simulink model "parkingValetVPP"  (R2023a)
settings: Solver=VariableStepAuto  StartTime=0.0  StopTime=Duration  RelTol=1e-3
values from neighbouring files (symbols this model uses):
  Duration = 15    [ParkingValetUsingNonlinearModelPredictiveControl1.m]
  egoTargetPose = [27.2,4.7,-pi/2]    [ParkingValetUsingNonlinearModelPredictiveControl1.m]
  pTracking = 10    [ParkingValetUsingNonlinearModelPredictiveControl1.m]
  tmax = tmin + 0.5    (= 5.5)    [ParkingValetUsingNonlinearModelPredictiveControl1.m]
  tmin = 5    [ParkingValetUsingNonlinearModelPredictiveControl1.m]
  Ts = 0.1    [ParkingValetUsingNonlinearModelPredictiveControl1.m]    (also in createMPCForTrackingVPP.m)
  TsPlanner = 1    [ParkingValetUsingNonlinearModelPredictiveControl1.m]
libraries: simulink x2, mpclib x1, robotmobilelib x1, mpcadaslib x1
settings Model: Creator=The MathWorks, Inc.  LastModifiedBy=The MathWorks, Inc.
settings SolverCC: MaxZcPerStep=1
settings OptimizationCC: ReuseModelBlockBuffer=off
settings ModelReferenceCC: EnableRefExpFcnMdlSchedulingChecks=on

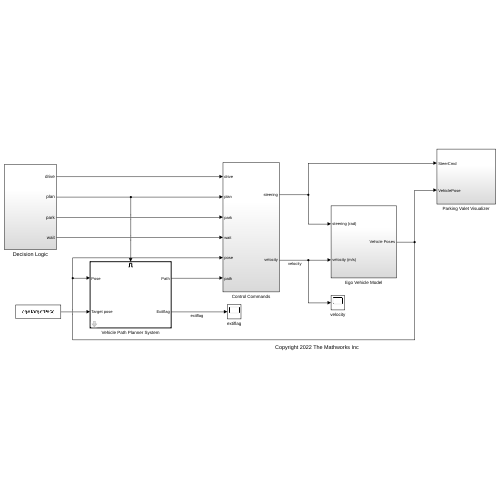
[thumbnail: Simulink's stored preview of the top-level diagram]
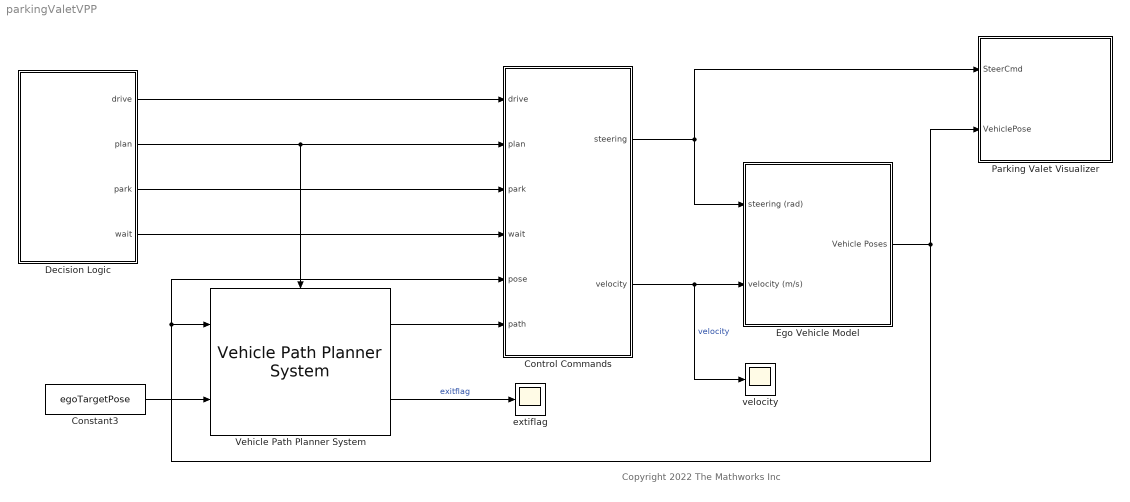
== system parkingValetVPP ==
  note: Copyright 2022 The Mathworks Inc
  Constant3 : Constant  Value=egoTargetPose
  Control Commands : Subsystem
  Decision Logic : Subsystem
  Ego Vehicle Model : Subsystem
  Parking Valet Visualizer : Subsystem
  Vehicle Path Planner System : mpcadaslib/Vehicle Path Planner System  egoLength=vdims.Length  egoWidth=vdims.Width  wheelbase=egoWheelbase  dist2Center=distToCenter  numObs=numObs  obsMat=obsMat  obs_ext=off  minDist=d_safe  Ts=TsPlanner  pPlanning=pPlanner  v_range=v_range  v_ext=off  steer_range=steer_range  steer_ext=off  suboptimal=off  maxiter=200  output_exitflag=on
      settings: LibrarySourceBlock=mpclib/Automated Driving/Vehicle Path Planner System
  extiflag : Scope
  velocity : Scope
  wires:
  Ego Vehicle Model/1(Vehicle Poses) -> Parking Valet Visualizer/2(VehiclePose), Control Commands/5(pose), Vehicle Path Planner System/1
  Control Commands/2(velocity) -> velocity/1, Ego Vehicle Model/2(velocity (m/s))  "velocity"
  Control Commands/1(steering) -> Ego Vehicle Model/1(steering (rad)), Parking Valet Visualizer/1(SteerCmd)
  Decision Logic/1(drive) -> Control Commands/1(drive)
  Decision Logic/2(plan) -> Vehicle Path Planner System/Enable, Control Commands/2(plan)
  Decision Logic/3(park) -> Control Commands/3(park)
  Decision Logic/4(wait) -> Control Commands/4(wait)
  Vehicle Path Planner System/1 -> Control Commands/6(path)
  Vehicle Path Planner System/2 -> extiflag/1  "exitflag"
  Constant3/1 -> Vehicle Path Planner System/2

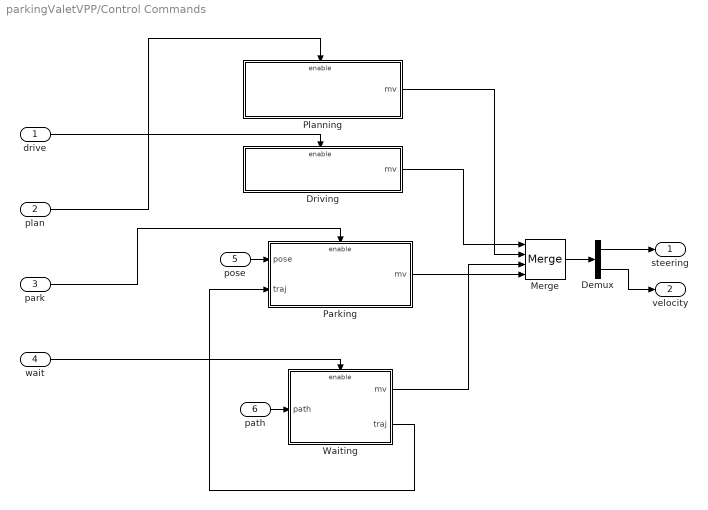
== system parkingValetVPP/Control Commands ==
  drive : Inport
  plan : Inport  Port=2
  park : Inport  Port=3
  wait : Inport  Port=4
  pose : Inport  Port=5
  path : Inport  Port=6
  Demux : Demux  Outputs=2
  Driving : Subsystem  TreatAsAtomicUnit=on
  Merge : Merge  Inputs=4
  "Parking " : Subsystem  TreatAsAtomicUnit=on
  Planning : Subsystem  TreatAsAtomicUnit=on
  Waiting : Subsystem  TreatAsAtomicUnit=on
  steering : Outport
  velocity : Outport  Port=2
  wires:
  "Parking "/1(mv) -> Merge/4
  Waiting/1(mv) -> Merge/3
  Merge/1 -> Demux/1
  Driving/1(mv) -> Merge/1
  pose/1 -> "Parking "/1(pose)
  drive/1 -> Driving/Enable
  Planning/1(mv) -> Merge/2
  Waiting/2(traj) -> "Parking "/2(traj)
  wait/1 -> Waiting/Enable
  path/1 -> Waiting/1(path)
  plan/1 -> Planning/Enable
  Demux/2 -> velocity/1
  park/1 -> "Parking "/Enable
  Demux/1 -> steering/1

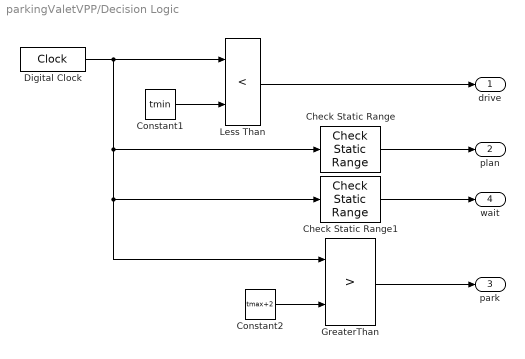
== system parkingValetVPP/Decision Logic ==
  Check Static Range : simulink/Model Verification/Check  Static Range  Description=tmin <= u <= tmax  max=tmax  max_included=on  min=tmin  min_included=on  enabled=off  stopWhenAssertionFail=off  export=on  icon=graphic
  Check Static Range1 : simulink/Model Verification/Check  Static Range  Description=tmax < u <= tmax+2  max=tmax+2  max_included=on  min=tmax  min_included=off  enabled=off  stopWhenAssertionFail=off  export=on  icon=graphic
  Constant1 : Constant  Value=tmin
  Constant2 : Constant  Value=tmax+2
  Digital Clock : DigitalClock  SampleTime=0.1
  GreaterThan : RelationalOperator  Operator=>  OutDataTypeStr=boolean  RndMeth=Simplest  InputSameDT=off
  Less Than : RelationalOperator  Operator=<  OutDataTypeStr=boolean  RndMeth=Simplest  InputSameDT=off
  drive : Outport
  plan : Outport  Port=2
  park : Outport  Port=3
  wait : Outport  Port=4
  wires:
  Constant1/1 -> Less Than/2
  Digital Clock/1 -> Check Static Range1/1, GreaterThan/1, Check Static Range/1, Less Than/1
  Constant2/1 -> GreaterThan/2
  GreaterThan/1 -> park/1
  Less Than/1 -> drive/1
  Check Static Range/1 -> plan/1
  Check Static Range1/1 -> wait/1

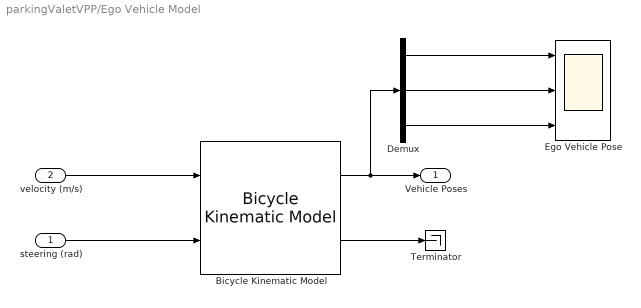
== system parkingValetVPP/Ego Vehicle Model ==
  steering (rad) : Inport
  velocity (m/s) : Inport  Port=2
  Bicycle Kinematic Model : robotmobilelib/Bicycle Kinematic Model  VehicleInputs=Vehicle Speed & Steering Angle  WheelBase=2.8  VehicleSpeedRange=[-6.5 6.5]  MaxSteeringAngle=pi/4  InitialState=egoInitialPose  SimulateUsing=Interpreted execution
  Demux : Demux  Outputs=3
  Ego Vehicle Pose : Scope  NumInputPorts=3
  Terminator : Terminator
  Vehicle Poses : Outport
  wires:
  Bicycle Kinematic Model/1 -> Demux/1, Vehicle Poses/1
  velocity (m/s)/1 -> Bicycle Kinematic Model/1
  steering (rad)/1 -> Bicycle Kinematic Model/2
  Bicycle Kinematic Model/2 -> Terminator/1
  Demux/3 -> Ego Vehicle Pose/3
  Demux/2 -> Ego Vehicle Pose/2
  Demux/1 -> Ego Vehicle Pose/1

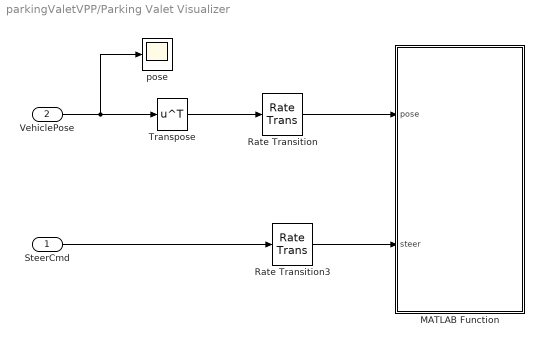
== system parkingValetVPP/Parking Valet Visualizer ==
  SteerCmd : Inport
  VehiclePose : Inport  Port=2
  MATLAB Function : MATLAB Function  TreatAsAtomicUnit=on
  Rate Transition : RateTransition  OutPortSampleTime=Tv
  Rate Transition3 : RateTransition  OutPortSampleTime=Tv
  Transpose : Math  Operator=transpose
  pose : Scope
  wires:
  Rate Transition/1 -> MATLAB Function/1(pose)
  VehiclePose/1 -> pose/1, Transpose/1
  Rate Transition3/1 -> MATLAB Function/2(steer)
  SteerCmd/1 -> Rate Transition3/1
  Transpose/1 -> Rate Transition/1

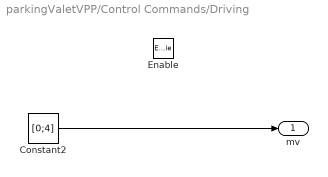
== system parkingValetVPP/Control Commands/Driving ==
  Enable : EnablePort  StatesWhenEnabling=reset
  Constant2 : Constant  Value=[0;4]  VectorParams1D=off
  mv : Outport
  wires:
  Constant2/1 -> mv/1

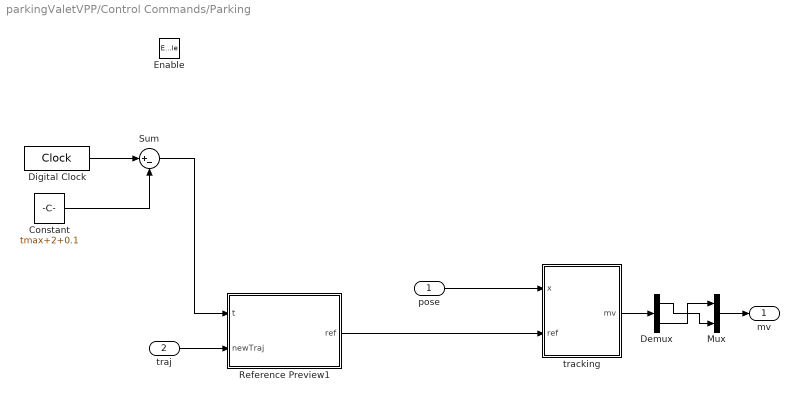
== system parkingValetVPP/Control Commands/Parking  ==
  pose : Inport
  traj : Inport  Port=2
  Enable : EnablePort  StatesWhenEnabling=reset
  Constant : Constant  Value=tmax+2+0.1
  Demux : Demux  Outputs=2
  Digital Clock : DigitalClock  SampleTime=0.1
  Mux : Mux  Inputs=2
  Reference Preview1 : MATLAB Function  TreatAsAtomicUnit=on
  Sum : Sum  Inputs=|+-
  tracking : Subsystem
  mv : Outport
  wires:
  Reference Preview1/1(ref) -> tracking/2(ref)
  pose/1 -> tracking/1(x)
  tracking/1(mv) -> Demux/1
  Demux/2 -> Mux/1
  Demux/1 -> Mux/2
  Mux/1 -> mv/1
  Sum/1 -> Reference Preview1/1(t)
  Digital Clock/1 -> Sum/1
  Constant/1 -> Sum/2
  traj/1 -> Reference Preview1/2(newTraj)

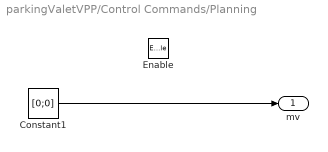
== system parkingValetVPP/Control Commands/Planning ==
  Enable : EnablePort  StatesWhenEnabling=reset
  Constant1 : Constant  Value=[0;0]  VectorParams1D=off
  mv : Outport
  wires:
  Constant1/1 -> mv/1

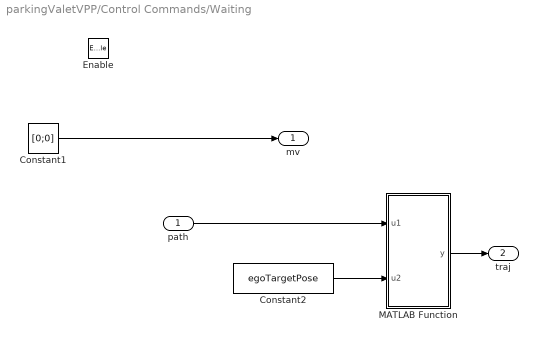
== system parkingValetVPP/Control Commands/Waiting ==
  path : Inport
  Enable : EnablePort  StatesWhenEnabling=reset
  Constant1 : Constant  Value=[0;0]  VectorParams1D=off
  Constant2 : Constant  Value=egoTargetPose
  MATLAB Function : MATLAB Function  TreatAsAtomicUnit=on
  mv : Outport
  traj : Outport  Port=2
  wires:
  Constant2/1 -> MATLAB Function/2(u2)
  path/1 -> MATLAB Function/1(u1)
  MATLAB Function/1(y) -> traj/1
  Constant1/1 -> mv/1

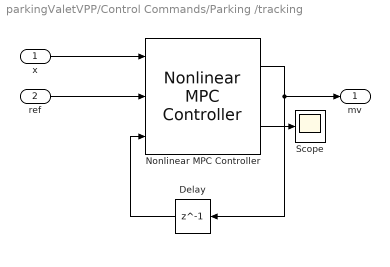
== system parkingValetVPP/Control Commands/Parking /tracking ==
  x : Inport
  ref : Inport  Port=2
  Delay : Delay  DelayLength=1
  Nonlinear MPC Controller : mpclib/Nonlinear MPC Controller  SCDEnableBlockLinearizationSpecification=on  nlmpcobj=nlobjTracking  UseObjectTs=on  UseMEX=off  mexname=''  md_enabled=off  mvtarget_enabled=off  param_enabled=off  cost_enabled=off  mvseq_enabled=off  stateseq_enabled=off  ovseq_enabled=off  slack_enabled=off  status_enabled=on  ov_min=off  ov_max=off  mv_min=off  mv_max=off  mvrate_min=off  mvrate_max=off  state_min=off  state_max=off  ov_weight=off  mv_weight=off  mvrate_weight=off  ecr_weight=off  nlp_initialize=off
  Scope : Scope
  mv : Outport
  wires:
  ref/1 -> Nonlinear MPC Controller/2
  Nonlinear MPC Controller/1 -> mv/1, Delay/1
  Delay/1 -> Nonlinear MPC Controller/3
  x/1 -> Nonlinear MPC Controller/1
  Nonlinear MPC Controller/2 -> Scope/1

== matlab function parkingValetVPP/Control Commands/Waiting/MATLAB Function ==
  data: u1 input; y output; u2 input; Duration parameter

function y = fcn(u1,u2, Duration)

traj = mpcInterpolatePathVPP(u1,u2,3,5);
Ts = 0.1;
%Duration = 25;
Tsteps = Duration/Ts;
y = [traj;repmat(traj(end,:),Tsteps-size(traj,1),1)];

== matlab function parkingValetVPP/Parking Valet Visualizer/MATLAB Function ==
  data: pose input; steer input; costmapStruct parameter
function visualizeParkingValet(pose, steer, costmapStruct)

%visualizePath Display simulation results.

coder.extrinsic('helperSLVisualizeParkingValet');

helperSLVisualizeParkingValet(pose, steer, costmapStruct);

== matlab function parkingValetVPP/Control Commands/Parking /Reference Preview1 ==
  data: t input; ref output; Ts parameter size=[1,1]; pTracking parameter size=[1,1]; Duration parameter size=[1,1]; newTraj input
function ref = fcn(t,Ts, pTracking, Duration, newTraj)
Tend = Duration;
T = t+(1:pTracking)*Ts;
T = min(T,Tend);
% Tsteps = Duration/Ts;
% p = length(traj)-1;
% Xref = [traj(2:p+1,:);repmat(traj(end,:),Tsteps-p,1)];
% time = Ts*(1:length(Xref));
% ref = interp1(time,Xref,T);

time = Ts*(1:length(newTraj));
ref = interp1(time,newTraj,T);
